simulink model "zynq_learn_ipcore"  (R2025b)
settings: Solver=FixedStepDiscrete  StartTime=0.0  StopTime=2e-06  FixedStep=2e-08  RelTol=1e-3
libraries: simulink x1
settings Model: DataTypeOverride=Off  Creator=kimsteph  LastModifiedBy=kimsteph
settings OptimizationCC: BlockReduction=off  ConditionallyExecuteInputs=off  DefaultParameterBehavior=Inlined  InheritOutputTypeSmallerThanSingle=on
settings DebuggingCC: ArtificialAlgebraicLoopMsg=error  SingleTaskRateTransMsg=error
settings HardwareCC: ProdBitPerPointer=32.0  ProdBitPerSizeT=32.0  ProdBitPerPtrDiffT=32.0  ProdLargestAtomicFloat=None  ProdIntDivRoundTo=Undefined  ProdEndianess=Unspecified  ProdWordSize=32.0  ProdHWDeviceType=ASIC/FPGA->ASIC/FPGA  TargetBitPerPointer=64.0  TargetBitPerSizeT=64.0  TargetBitPerPtrDiffT=64.0  TargetLongLongMode=on  TargetIntDivRoundTo=Zero  TargetEndianess=LittleEndian  TargetWordSize=64.0  TargetHWDeviceType=Custom Processor->MATLAB Host Computer  ProdEqTarget=off

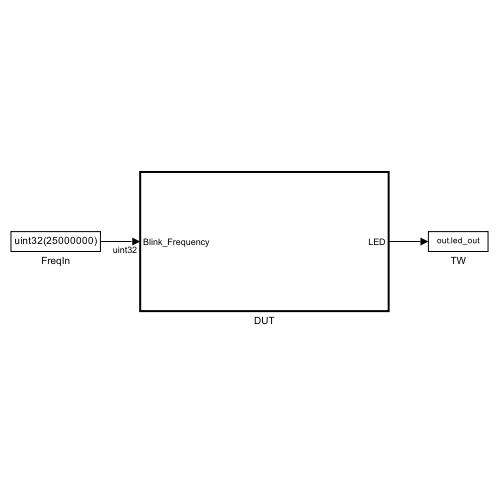
[thumbnail: Simulink's stored preview of the top-level diagram]
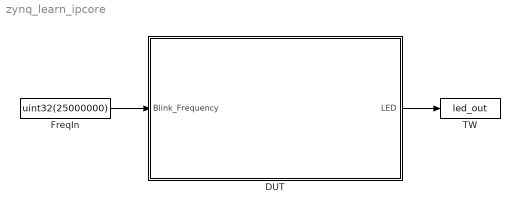
== system zynq_learn_ipcore ==
  DUT : Subsystem  TreatAsAtomicUnit=on
  FreqIn : Constant  Value=uint32(25000000)  OutDataTypeStr=uint32
  TW : ToWorkspace  VariableName=led_out  SaveFormat=Timeseries  SampleTime=-1
  wires:
  FreqIn/1 -> DUT/1(Blink_Frequency)
  DUT/1(LED) -> TW/1

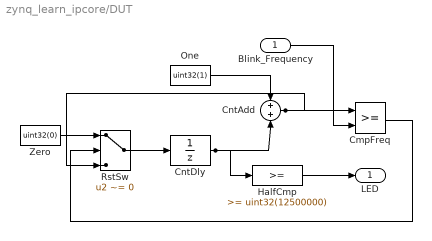
== system zynq_learn_ipcore/DUT ==
  Blink_Frequency : Inport  OutDataTypeStr=uint32
  CmpFreq : RelationalOperator  OutDataTypeStr=boolean  RndMeth=Simplest  InputSameDT=off
  CntAdd : Sum  OutDataTypeStr=uint32
  CntDly : UnitDelay  SampleTime=2e-08  HasFrameUpgradeWarning=on
  HalfCmp : simulink/Logic and Bit Operations/Compare To Constant  relop=>=  const=uint32(12500000)  OutDataTypeStr=boolean
  One : Constant  Value=uint32(1)  OutDataTypeStr=uint32
  RstSw : Switch  Criteria=u2 ~= 0  SaturateOnIntegerOverflow=off  InputSameDT=off
  Zero : Constant  Value=uint32(0)  OutDataTypeStr=uint32
  LED : Outport
  wires:
  CmpFreq/1 -> RstSw/2
  One/1 -> CntAdd/1
  Zero/1 -> RstSw/1
  CntDly/1 -> CntAdd/2, HalfCmp/1
  RstSw/1 -> CntDly/1
  Blink_Frequency/1 -> CmpFreq/2
  CntAdd/1 -> CmpFreq/1, RstSw/3
  HalfCmp/1 -> LED/1
